simulink model "WPL_APA_parallel"  (R2020b)
settings: Solver=FixedStepAuto  StartTime=0.0  StopTime=inf  FixedStep=0.02  RelTol=1e-3
undefined symbols (not defined in the file): Drive, Steer
libraries: robotlib x10, simulink x1
(part 1 of 3)
settings Model: Creator=DwigHT  LastModifiedBy=DwigHT
settings OptimizationCC: EnhancedBackFolding=on  PassReuseOutputArgsAs=Individual arguments  ZeroExternalMemoryAtStartup=off  ZeroInternalMemoryAtStartup=off  MaxStackSize=64  OptimizeBlockOrder=speed  DifferentSizesBufferReuse=on  OptimizationCustomize=off  EfficientTunableParamExpr=on
settings DebuggingCC: ParameterTunabilityLossMsg=error
settings HardwareCC: ProdBitPerPointer=32  ProdBitPerSizeT=32  ProdBitPerPtrDiffT=32  ProdLargestAtomicFloat=None  ProdIntDivRoundTo=Undefined  ProdEndianess=Unspecified  ProdWordSize=32  ProdHWDeviceType=Generic->Unspecified (assume 32-bit Generic)
settings SFSimCC: MATLABDynamicMemAlloc=off
settings RTWCC: Description=Embedded Coder  SystemTargetFile=ert.tlc  HardwareBoard=Robot Operating System (ROS)  TLCOptions="-aInlineSetEventsForThisBaseRateFcn=TLC_FALSE -aSuppressMultiTaskScheduler=TLC_FALSE  -aRateBasedStepFcn=0"  TemplateMakefile=ert_default_tmf  Toolchain=Catkin  TargetLang=C++
settings CodeAppCC: ForceParamTrailComments=on  IgnoreCustomStorageClasses=off  OperatorAnnotations=on  SimulinkDataObjDesc=on  SFDataObjDesc=on  InsertBlockDesc=on
settings ERTTargetCC: SupportVariableSizeSignals=on

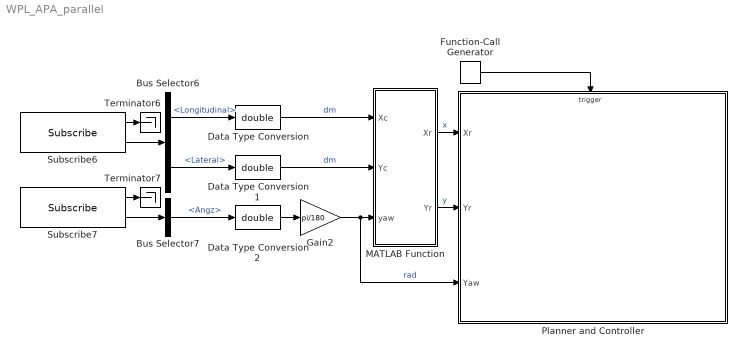
== system WPL_APA_parallel ==
  Bus Selector6 : BusSelector  OutputSignals=Longitudinal,Lateral
  Bus Selector7 : BusSelector  OutputSignals=Angz
  Data Type Conversion : DataTypeConversion  OutDataTypeStr=double
  Data Type Conversion1 : DataTypeConversion  OutDataTypeStr=double
  Data Type Conversion2 : DataTypeConversion  OutDataTypeStr=double
  Function-Call Generator : simulink/Ports & Subsystems/Function-Call Generator  sample_time=0.1  numberOfIterations=1  DisallowWideOutput=off
  Gain2 : Gain  Gain=pi/180
  MATLAB Function : MATLAB Function  TreatAsAtomicUnit=on
  Planner and Controller : Subsystem
  Subscribe6 : robotlib/Subscribe  topicSource=Select from ROS network  topic=/WPL_pos  messageType=WPLpos_msgs/WPLpos  SampleTime=-1  legacyBusStruct=off  messageQueueLength=1
  Subscribe7 : robotlib/Subscribe  topicSource=Select from ROS network  topic=/imu_info  messageType=WPLimu_msgs/WPLimu  SampleTime=-1  legacyBusStruct=off  messageQueueLength=1
  Terminator6 : Terminator
  Terminator7 : Terminator
  wires:
  Subscribe6/1 -> Terminator6/1
  Bus Selector7/1 -> Data Type Conversion2/1  "<Angz>"
  Subscribe7/2 -> Bus Selector7/1
  Subscribe6/2 -> Bus Selector6/1
  Subscribe7/1 -> Terminator7/1
  Bus Selector6/1 -> Data Type Conversion/1  "<Longitudinal>"
  Function-Call Generator/1 -> Planner and Controller/Trigger
  MATLAB Function/1(Xr) -> Planner and Controller/1(Xr)  "x"
  MATLAB Function/2(Yr) -> Planner and Controller/2(Yr)  "y"
  Bus Selector6/2 -> Data Type Conversion1/1  "<Lateral>"
  Data Type Conversion/1 -> MATLAB Function/1(Xc)  "dm"
  Data Type Conversion1/1 -> MATLAB Function/2(Yc)  "dm"
  Gain2/1 -> Planner and Controller/3(Yaw), MATLAB Function/3(yaw)  "rad"
  Data Type Conversion2/1 -> Gain2/1

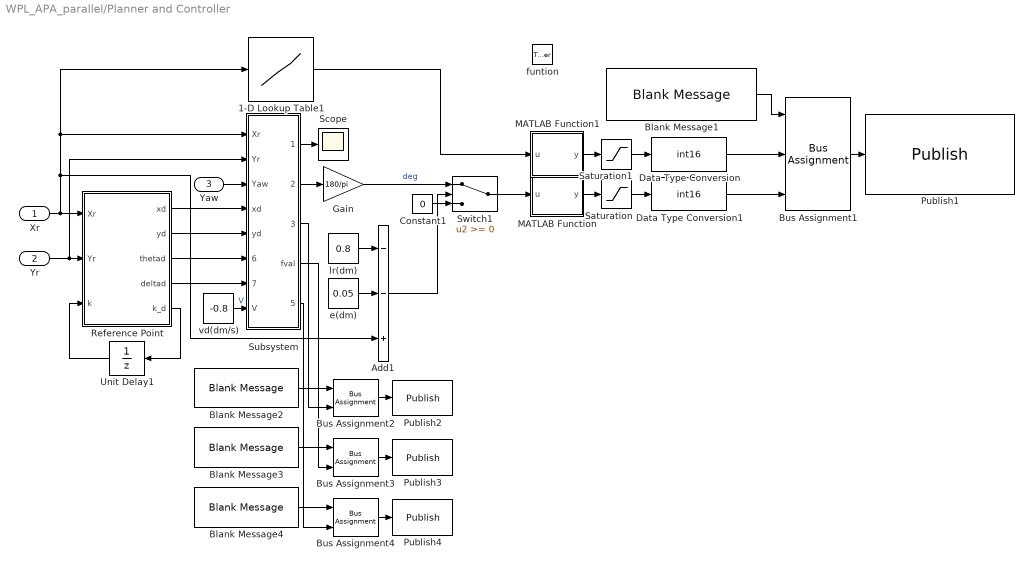
== system WPL_APA_parallel/Planner and Controller ==
  Xr : Inport
  Yr : Inport  Port=2
  Yaw : Inport  Port=3
  funtion : TriggerPort  TriggerType=function-call  VariantControl=Variant
  1-D Lookup Table1 : Lookup_n-D  NumberOfTableDimensions=1  BreakpointsForDimension1=[0 0.05 0.3 2.6 7.5 7.6 8]  Table=[2048 2048 2300 2400 2400 2400 2400]  InternalRulePriority=Speed  RndMeth=Simplest  InputSameDT=on
  Add1 : Sum  Inputs=--+
  Blank Message1 : robotlib/Blank Message  messageClass=Message  entityType=WPLchassis_msgs/WPLch  messageType=WPLchassis_msgs/WPLch  SampleTime=inf  legacyBusStruct=off
  Blank Message2 : robotlib/Blank Message  messageClass=Message  entityType=std_msgs/Float64  messageType=std_msgs/Float64  SampleTime=inf  legacyBusStruct=off
  Blank Message3 : robotlib/Blank Message  messageClass=Message  entityType=std_msgs/Float64  messageType=std_msgs/Float64  SampleTime=inf  legacyBusStruct=off
  Blank Message4 : robotlib/Blank Message  messageClass=Message  entityType=std_msgs/Float64  messageType=std_msgs/Float64  SampleTime=inf  legacyBusStruct=off
  Bus Assignment1 : BusAssignment  AssignedSignals=Drive,Steer
  Bus Assignment2 : BusAssignment  AssignedSignals=Data
  Bus Assignment3 : BusAssignment  AssignedSignals=Data
  Bus Assignment4 : BusAssignment  AssignedSignals=Data
  Constant1 : Constant  Value=0
  Data Type Conversion : DataTypeConversion  OutDataTypeStr=int16
  Data Type Conversion1 : DataTypeConversion  OutDataTypeStr=int16
  Gain : Gain  Gain=180/pi
  MATLAB Function : MATLAB Function  TreatAsAtomicUnit=on
  MATLAB Function1 : MATLAB Function  TreatAsAtomicUnit=on
  Publish1 : robotlib/Publish  topicSource=Select from ROS network  topic=/control_info  messageType=WPLchassis_msgs/WPLch  legacyBusStruct=off  messageQueueLength=1
  Publish2 : robotlib/Publish  topicSource=Specify your own  topic=/delta_t  messageType=std_msgs/Float64  legacyBusStruct=off  messageQueueLength=1
  Publish3 : robotlib/Publish  topicSource=Specify your own  topic=/fval  messageType=std_msgs/Float64  legacyBusStruct=off  messageQueueLength=1
  Publish4 : robotlib/Publish  topicSource=Specify your own  topic=/exitflag  messageType=std_msgs/Float64  legacyBusStruct=off  messageQueueLength=1
  Reference Point : MATLAB Function  TreatAsAtomicUnit=on
  Saturation : Saturate  UpperLimit=4095  LowerLimit=0
  Saturation1 : Saturate  UpperLimit=4095  LowerLimit=0
  Scope : Scope
  Subsystem : Subsystem
  Switch1 : Switch
  Unit Delay1 : UnitDelay  InitialCondition=1  SampleTime=-1  HasFrameUpgradeWarning=on
  e(dm) : Constant  Value=0.05
  lr(dm) : Constant  Value=0.8
  vd(dm/s) : Constant  Value=-0.8
  wires:
  Reference Point/2(yd) -> Subsystem/5(yd)
  vd(dm/s)/1 -> Subsystem/8(V)  "V"
  Reference Point/4(deltad) -> Subsystem/7(deltad)
  Reference Point/3(thetad) -> Subsystem/6(thetad)
  Unit Delay1/1 -> Reference Point/3(k)
  Reference Point/1(xd) -> Subsystem/4(xd)
  Reference Point/5(k_d) -> Unit Delay1/1
  Gain/1 -> Switch1/1  "deg"
  Xr/1 -> Add1/3, 1-D Lookup Table1/1, Subsystem/1(Xr), Reference Point/1(Xr)
  Yr/1 -> Subsystem/2(Yr), Reference Point/2(Yr)
  Subsystem/1(v_des) -> Scope/1
  Subsystem/2(delta_des) -> Gain/1
  Constant1/1 -> Switch1/3
  Add1/1 -> Switch1/2
  Subsystem/3(delta_t) -> Bus Assignment2/2
  Subsystem/4(fval) -> Bus Assignment3/2
  Subsystem/5(exitflag) -> Bus Assignment4/2
  Yaw/1 -> Subsystem/3(Yaw)
  Bus Assignment4/1 -> Publish4/1
  Blank Message3/1 -> Bus Assignment3/1
  Bus Assignment3/1 -> Publish3/1
  Blank Message4/1 -> Bus Assignment4/1
  Blank Message2/1 -> Bus Assignment2/1
  Bus Assignment2/1 -> Publish2/1
  Data Type Conversion1/1 -> Bus Assignment1/3
  Data Type Conversion/1 -> Bus Assignment1/2
  Bus Assignment1/1 -> Publish1/1
  Blank Message1/1 -> Bus Assignment1/1
  Switch1/1 -> MATLAB Function/1(u)
  lr(dm)/1 -> Add1/1
  e(dm)/1 -> Add1/2
  Saturation/1 -> Data Type Conversion1/1
  MATLAB Function/1(y) -> Saturation/1
  MATLAB Function1/1(y) -> Saturation1/1
  Saturation1/1 -> Data Type Conversion/1
  1-D Lookup Table1/1 -> MATLAB Function1/1(u)

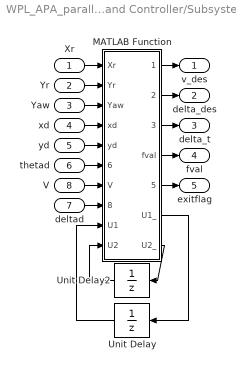
== system WPL_APA_parallel/Planner and Controller/Subsystem ==
  Xr : Inport
  Yr : Inport  Port=2
  Yaw : Inport  Port=3
  xd : Inport  Port=4
  yd : Inport  Port=5
  thetad : Inport  Port=6
  deltad : Inport  Port=7
  V : Inport  Port=8
  MATLAB Function : MATLAB Function  TreatAsAtomicUnit=on
  Unit Delay : UnitDelay  SampleTime=-1  HasFrameUpgradeWarning=on
  Unit Delay2 : UnitDelay  SampleTime=-1  HasFrameUpgradeWarning=on
  v_des : Outport
  delta_des : Outport  Port=2
  delta_t : Outport  Port=3
  fval : Outport  Port=4
  exitflag : Outport  Port=5
  wires:
  Unit Delay/1 -> MATLAB Function/9(U1)
  MATLAB Function/7(U2_) -> Unit Delay2/1
  Unit Delay2/1 -> MATLAB Function/10(U2)
  Yr/1 -> MATLAB Function/2(Yr)
  yd/1 -> MATLAB Function/5(yd)
  MATLAB Function/6(U1_) -> Unit Delay/1
  xd/1 -> MATLAB Function/4(xd)
  V/1 -> MATLAB Function/7(V)
  MATLAB Function/1(v_des) -> v_des/1
  Xr/1 -> MATLAB Function/1(Xr)
  Yaw/1 -> MATLAB Function/3(Yaw)
  thetad/1 -> MATLAB Function/6(thetad)
  MATLAB Function/2(delta_des) -> delta_des/1
  deltad/1 -> MATLAB Function/8(deltad)
  MATLAB Function/3(delta_t) -> delta_t/1
  MATLAB Function/4(fval) -> fval/1
  MATLAB Function/5(exitflag) -> exitflag/1

== matlab function WPL_APA_parallel/Planner and Controller/MATLAB Function ==
  data: u input; y output
function y = fcn(u)
if u<0
    u=u/30*1800+2000;
else
    u=u/30*1200+2200;
end
y = round(u);

== matlab function WPL_APA_parallel/MATLAB Function ==
  data: Xc input; Xr output; Yc input; yaw input; Yr output
function [Xr,Yr] = fcn(Xc,Yc,yaw)
lr=0.85;
Xr=Xc-lr*cos(yaw);
Yr=Yc-lr*sin(yaw);
